simulink model "LGS_allFaultStuffDeleted"  (R2019b)
settings: Solver=FixedStepDiscrete  StartTime=0.0  StopTime=45.0  FixedStep=0.1  RelTol=1e-3
model workspace (MAT data in the model file):
  fipData : object (value not decoded)
  fipName : object (value not decoded)
  stepSize = 0.1
libraries: commrandsrc3 x16, simulink x3, LibFailureCondition x1
(part 7 of 7)

== stateflow chart LGS_allFaultStuffDeleted/Digital Part/Computing module1/RetractionSequence ==
  state CloseGeneralValve
    entry: GeneralValve = false;
    entry: stateNumber =int8(6);
  state Idle
    entry: GeneralValve = false;
    entry: OpenDoorValve = false;
    entry: GearRetractionValve = false;
    entry: CloseDoorValve = false;
    entry: stateNumber = int8(0);
  state stimulateGeneralValve
    entry: GeneralValve = true;
    entry: stateNumber = int8(1);
  state InterruptDetected
    entry: GeneralValve = true;
  state StopStimulatingCloseDoorValve
    entry: CloseDoorValve = false;
    entry: stateNumber = int8(5);
  state StimulateOpenDoorValve
    entry: OpenDoorValve = true;
    entry: CloseDoorValve = false;
    entry: stateNumber = int8(2);
  state Interruption
    entry: GearRetractionValve = false;
  state StopGRVandODVstartCDV
    entry: GearRetractionValve = false;
    entry: OpenDoorValve = false;
    entry: CloseDoorValve = true;
    entry: stateNumber = int8(4);
  state StimulateGearRetractionValve
    entry: GearRetractionValve = true;
    entry: stateNumber = int8(3);
  (default) -> Idle
  CloseGeneralValve -> Idle [order 1] : [(~ExtensionInterruption)]
  InterruptDetected -> CloseGeneralValve [order 5] : [(InterruptStateNo == 1)]
  Idle -> InterruptDetected [order 2] : [((InterruptStateNo ~=0) && (StartRetractionSequence))]
  CloseGeneralValve -> Interruption [order 2] : [(ExtensionInterruption)]
  StopStimulatingCloseDoorValve -> CloseGeneralValve [order 1] : [(~ExtensionInterruption)]
  Idle -> stimulateGeneralValve [order 1] : [((((StartRetractionSequence) && (AllDoorsLockedClosed)) && (AllGearsLockedDown)) && (InterruptStateNo == 0))]
  Interruption -> Idle
  InterruptDetected -> stimulateGeneralValve [order 1] : [(InterruptStateNo == 6)]
  InterruptDetected -> StimulateOpenDoorValve [order 4] : [((InterruptStateNo == 4) || (InterruptStateNo == 5))]
  InterruptDetected -> StopGRVandODVstartCDV [order 2] : [(InterruptStateNo == 2)]
  InterruptDetected -> StimulateGearRetractionValve [order 3] : [(InterruptStateNo == 3)]
  stimulateGeneralValve -> StimulateOpenDoorValve [order 1] : [(~ExtensionInterruption)]
  stimulateGeneralValve -> Interruption [order 2] : [(ExtensionInterruption)]
  StopStimulatingCloseDoorValve -> Interruption [order 2] : [(ExtensionInterruption)]
  StopGRVandODVstartCDV -> StopStimulatingCloseDoorValve [order 1] : [((AllDoorsLockedClosed) && (~ExtensionInterruption))]
  StopGRVandODVstartCDV -> Interruption [order 2] : [(ExtensionInterruption)]
  StimulateOpenDoorValve -> Interruption [order 2] : [(ExtensionInterruption)]
  StimulateGearRetractionValve -> Interruption [order 2] : [(ExtensionInterruption)]
  StimulateOpenDoorValve -> StimulateGearRetractionValve [order 1] : [(((AllDoorsOpened) && (AllShockAbsorbersRelaxed)) && (~ExtensionInterruption))]
  StimulateOpenDoorValve -> StopGRVandODVstartCDV [order 3] : [(((AllDoorsOpened) && (~AllShockAbsorbersRelaxed)) && (~ExtensionInterruption))]
  StimulateGearRetractionValve -> StopGRVandODVstartCDV [order 1] : [((AllGearsLockedUp) && (~ExtensionInterruption))]
  data: StartRetractionSequence input boolean; GeneralValve output boolean; OpenDoorValve output boolean; AllDoorsOpened input boolean; AllDoorsLockedClosed input boolean; AllGearsLockedDown input boolean; AllGearsLockedUp input boolean; CloseDoorValve output boolean; AllShockAbsorbersRelaxed input boolean [0..3]; ExtensionInterruption input boolean; GearRetractionValve output boolean; InterruptStateNo input int8 [0..6]; stateNumber output int8 [0..6]

== stateflow chart LGS_allFaultStuffDeleted/FailureConditionObserver/FC2/FC_FC2_output/Chart ==
  state handleIsUp
    en: out = true;
  state handleIsDown
    en: time = int8(149);
    en: out = true;
    du: time = time - 1;
  state gearIsNotDown
    en: out = false;
  state gearIsDown
    en: out = true;
  (default) -> handleIsUp
  gearIsNotDown -> handleIsUp : [(handleUp)]
  gearIsDown -> handleIsUp : [(handleUp)]
  handleIsUp -> handleIsDown : [(~(handleUp))]
  handleIsDown -> handleIsUp [order 1] : [(handleUp)]
  handleIsDown -> gearIsNotDown [order 3] : [(time==0)]
  handleIsDown -> gearIsDown [order 2] : [(gearDown)]
  data: out output boolean; handleUp input boolean; time local int8 [0..150]; gearDown input boolean
